simulink library "sm_carousel_lib"  (R2021b)
settings: Solver=ode45  StartTime=0.0  StopTime=10.0  RelTol=1e-3  EnableMultiTasking=on
undefined symbols (not defined in the file): X, Y, Z
libraries: sm_lib x123, $bdroot x16, fl_lib x12, nesl_utility x2
(part 1 of 4)
settings Model: Creator=The MathWorks, Inc.  LastModifiedBy=The MathWorks, Inc.
settings SolverCC: AlgebraicLoopSolver=TrustRegion
settings DataIOCC: LimitDataPoints=on  SaveFormat=Array  ReturnWorkspaceOutputs=off
settings OptimizationCC: ExpressionDepthLimit=2147483647  LifeSpan=inf
settings DebuggingCC: UnderspecifiedInitializationDetection=Classic  MergeDetectMultiDrivingBlocksExec=none  SolverPrmCheckMsg=warning  StateNameClashWarn=warning  SFUnexpectedBacktrackingDiag=warning  SFNoUnconditionalDefaultTransitionDiag=warning  SFExecutionAtInitializationDiag=none  SFMachineParentedDataDiag=warning  ArithmeticOperatorsInVariantConditions=warning
settings HardwareCC: ProdBitPerPointer=32  ProdBitPerSizeT=32  ProdBitPerPtrDiffT=32  ProdLargestAtomicFloat=None  ProdIntDivRoundTo=Undefined  ProdEndianess=Unspecified  ProdWordSize=32  ProdHWDeviceType=32-bit Generic
settings ModelReferenceCC: PropagateSignalLabelsOutOfModel=off
settings SFSimCC: SimUseLocalCustomCode=off  CustomCodeUndefinedFunction=UseInterfaceOnly
settings RTWCC: RTWUseLocalCustomCode=off
settings CodeAppCC: StateflowObjectComments=on
settings GRTTargetCC: TargetLangStandard=C89/C90 (ANSI)
settings ConfigComp: CovMetricSettings=dw  CovSaveCumulativeToWorkspaceVar=on  CovSaveSingleToWorkspaceVar=on  CovExternalEMLEnable=off  CovSFcnEnable=off

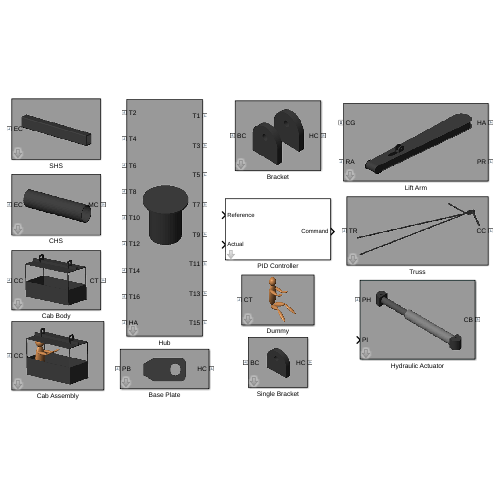
[thumbnail: Simulink's stored preview of the top-level diagram]
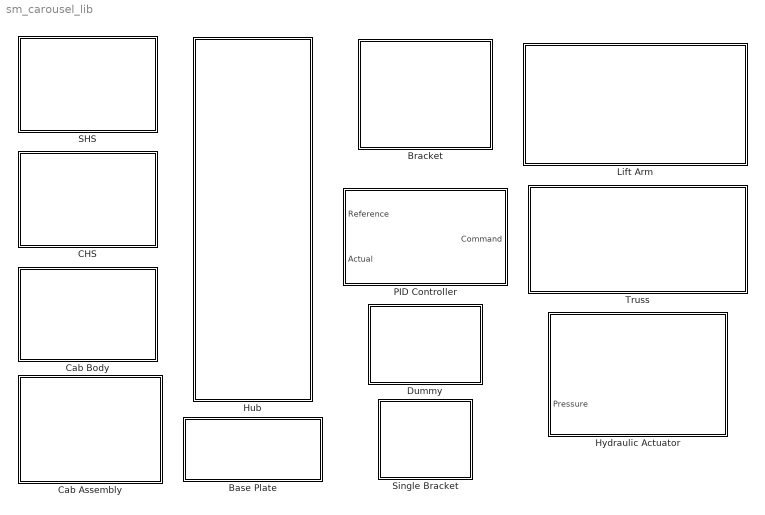
== system sm_carousel_lib ==
  Base Plate : Subsystem  mask(Base Plate){ConnectionDepth=0.1, BasePlateWidth=0.4, BasePlateHeight=0.2, TaperedLength=0.1, rHole=0.05, BasePlateThickness=0.01, HoleOffset=0.3, rho=7800, PlateColor=[0.3 0.3 0.3]}
      mask prompts: ConnectionDepth "Connection Depth (m)"; BasePlateWidth "Plate Width (m)"; BasePlateHeight "Plate Height (m)"; TaperedLength "Tapered Length (m)"; rHole "Hole Radius (m)"; BasePlateThickness "Plate Thickness (m)"; HoleOffset "Hole Offset (m)"; rho "Density (kg/m^3)"; PlateColor "Color [r g b]"
      mask help:
      | This block models a structural element called a Base Plate.
      |
      | It is a utility part designed to serve two purposes:
      | 1) Provide a method to connect the Cab Assembly to the truss via a revolute.
      | 2) To connect the CHS and SHS elements in the Truss block.
      |
      | Attachment points are:
      | 1) The central point of the cross-section at one end of the element (PB).
      | 2) The center of the hole (HC).
      |
      | Click on Help to view a schematic of the Base Plate and its configurable dimension parameters.
      mask init:
      | points = 40;
      | 
      | thetaHole = linspace(pi,-pi,points);
      | 
      | hole = [rHole*cos(thetaHole)+HoleOffset;...
      |     rHole*sin(thetaHole)]';
      | 
      | outerVertices = [0 0;...
      |     0 -0.5*ConnectionDepth;...
      |     TaperedLength -0.5*BasePlateHeight;...
      |     BasePlateWidth -0.5*BasePlateHeight;...
      |     BasePlateWidth 0.5*BasePlateHeight;...
      |     TaperedLength 0.5*BasePlateHeight;...
      |     0 0.5*ConnectionDepth;
      |     0 0];
      |     
      | outer = simmechanics.demohelpers.round_corners(outerVertices,[4 5],rHole,points);
      | 
      | BasePlatePoints = [hole;outer];
      mask Help: web(fullfile(matlabroot,'toolbox','physmod','sm','smdemos','carousel','demohelp','sm_carousel_base_plate.html'));
      mask DialogControl Tab01 Prompt: Dimensions
      mask DialogControl Tab02 Prompt: Material Properties
      mask Display:
      | image(fullfile(matlabroot,'toolbox','physmod','sm','smdemos','carousel','images','sm_carousel_base_plate.png'));
      | port_label('lconn',1,'PB');
      | port_label('rconn',1,'HC');
  Bracket : Subsystem  mask(Bracket){Hbracket=0.75, Wbracket=0.75, Tbracket=0.15, Dbracket=0.8, Hhole=0.5, Rhole=0.075, rhoBracket=7800, bracketColor=[0.3 0.3 0.3]}
      mask prompts: Hbracket "Hbracket (m)"; Wbracket "Wbracket (m)"; Tbracket "Tbracket (m)"; Dbracket "Dbracket (m)"; Hhole "Hhole (m)"; Rhole "Rhole (m)"; rhoBracket "Density (kg/m^3)"; bracketColor "Bracket Color [r g b]"
      mask help:
      | This block models a double-sided bracket.
      |
      | Attachment points are:
      | 1) The base of the bracket centered between the two elements (BC).
      | 2) The central point between the two holes which is configured for Revolute joints (HC).
      |
      | Click on Help to view a schematic of the bracket and its configurable dimension parameters.
      mask init:
      | points = 40;
      | 
      | y = Hbracket - (Wbracket/2);
      | 
      | outerVertices = [0 0;...
      |     Wbracket/2 0;...
      |     Wbracket/2 y;...
      |     Wbracket/2 Hbracket;...
      |     -Wbracket/2 Hbracket;...
      |     -Wbracket/2 y;...
      |     -Wbracket/2 0;...
      |     0 0];
      | 
      | outer = simmechanics.demohelpers.round_corners(outerVertices,[4 5],Wbracket/2,points);
      | 
      | thetaHole = linspace(1.5*pi,-0.5*pi,points);
      | hole = [Rhole*cos(thetaHole);...
      |     Rhole*sin(thetaHole)+Hhole]';
      | 
      | bracketPoints = [hole;outer];
      mask Help: web(fullfile(matlabroot,'toolbox','physmod','sm','smdemos','carousel','demohelp','sm_carousel_bracket.html'));
      mask DialogControl Tab01 Prompt: Dimensions
      mask DialogControl Tab02 Prompt: Material Properties
      mask Display:
      | image(fullfile(matlabroot,'toolbox','physmod','sm','smdemos','carousel','images','sm_carousel_bracket.png'));
      | port_label('lconn',1,'BC');
      | port_label('rconn',1,'HC');
  CHS : Subsystem  mask(Circular Hollow Section (CHS)){PinOuterRadius=0.1, PinThickness=0.01, PinDepth=1, rhoPin=7800, PinColor=[0.3 0.3 0.3]}
      mask prompts: PinOuterRadius "Outer Radius (m)"; PinThickness "Thickness (m)"; PinDepth "Length (m)"; rhoPin "Density (kg/m^3)"; PinColor "Color [r g b]"
      mask help:
      | This block models a Circular Hollow Section structural element.
      |
      | Attachment points are:
      | 1) The central point of the cross-section at one end of the element (EC).
      | 2) The central point of the cross-section at the center of the element (MC).
      |
      | Click on Help to view a schematic of the CHS and its configurable dimension parameters.
      mask init:
      | %%% Pin
      | 
      | points = 40;
      | 
      | PinInnerRadius = PinOuterRadius-PinThickness;
      | 
      | thetaInner = linspace(2*pi,0,points);
      | inner = [PinInnerRadius*cos(thetaInner);...
      |     PinInnerRadius*sin(thetaInner)]';
      | 
      | thetaOuter = fliplr(thetaInner);
      | outer = [PinOuterRadius*cos(thetaOuter);...
      |     PinOuterRadius*sin(thetaOuter)]';
      | 
      | Pin = [inner;outer];
      | 
      | %%% End Pin
      mask Help: web(fullfile(matlabroot,'toolbox','physmod','sm','smdemos','carousel','demohelp','sm_carousel_CHS.html'));
      mask DialogControl Tab01 Prompt: Dimensions
      mask DialogControl Tab02 Prompt: Material Properties
      mask Display:
      | image(fullfile(matlabroot,'toolbox','physmod','sm','smdemos','carousel','images','sm_carousel_CHS.png'));
      | port_label('lconn',1,'EC');
      | port_label('rconn',1,'MC');
  Cab Assembly : Subsystem  mask(Cab Assembly){CabLength=1.5, CabWidth=0.75, CabPlateThickness=0.02, CabBodyConnW=0.05, CabBodyConnH=0.07, CabWindowHeight=0.5, SpacerThickness=0.02, CabTubDepth=0.45, RP_CD=0.1, RP_W=0.23, RP_H=0.18, RP_TL=0.07, RP_HR=0.04, RP_PT=0.01, RP_HO=0.15, DummyHeight=1.83, DummyDensity=950, rhoCab=7800, CabColor=[0.3 0.3 0.3]}
      mask prompts: CabLength "Cab Length (m)"; CabWidth "Cab Width (m)"; CabPlateThickness "Cab Plate Thickness (m)"; CabBodyConnW "Cab Body Connector Width (m)"; CabBodyConnH "Cab Body Connector Height (m)"; CabWindowHeight "Cab Window Height (m)"; SpacerThickness "Cab Window Column Thickness (m)"; CabTubDepth "Cab Tub Depth (m)"; RP_CD "Connection Depth (m)"; RP_W "Plate Width (m)"; RP_H "Plate Height (m)"; RP_TL "Tapered Length (m)"; RP_HR "Hole Radius (m)"; RP_PT "Plate Thickness (m)"; RP_HO "Hole Offset (m)"; DummyHeight "Dummy Height (m)"; DummyDensity "Dummy Density (kg/m^3)"; rhoCab "Cab Density (kg/m^3)"; CabColor "Cab Color [r g b]"
      mask help:
      | This block models the Carousel Cab Assembly.
      |
      | The block includes: 2x Base Plate, 1x Cab Body, 1x Dummy.
      |
      | Attachment point is the central point between the holes of the two revolute plates.
      |
      | Click on Help to view a schematic of the Cab Assembly. The configurable dimensions are not shown. Refer to the Help of the individual parts for more information.
      mask Help: web(fullfile(matlabroot,'toolbox','physmod','sm','smdemos','carousel','demohelp','sm_carousel_cab_assembly.html'));
      mask DialogControl Tab01 Prompt: Cab Body Main
      mask DialogControl Tab02 Prompt: Cab Body Revolute Plate
      mask DialogControl Tab03 Prompt: Dummy
      mask DialogControl Tab04 Prompt: Material Properties
      mask Display:
      | image(fullfile(matlabroot,'toolbox','physmod','sm','smdemos','carousel','images','sm_carousel_cab_assembly.png'));
      | port_label('lconn',1,'CC');
  Cab Body : Subsystem  mask(Cab Body){CabLength=1.5, CabWidth=0.75, PlateThickness=0.02, ConnectorWidth=0.05, ConnectorHeight=0.07, SpacerHeight=0.5, SpacerThickness=0.02, TubDepth=0.45, RP_CD=0.1, RP_W=0.23, RP_H=0.18, RP_TL=0.07, RP_HR=0.04, RP_PT=0.01, RP_HO=0.15, rhoCab=7800, CabColor=[0.3 0.3 0.3]}
      mask prompts: CabLength "Cab Length (m)"; CabWidth "Cab Width (m)"; PlateThickness "Cab Plate Thickness (m)"; ConnectorWidth "Connector Width (m)"; ConnectorHeight "Connector Height (m)"; SpacerHeight "Spacer Height (m)"; SpacerThickness "Spacer Thickness (m)"; TubDepth "Tub Depth (m)"; RP_CD "Connection Depth (m)"; RP_W "Plate Width (m)"; RP_H "Plate Height (m)"; RP_TL "Tapered Length (m)"; RP_HR "Hole Radius (m)"; RP_PT "Plate Thickness (m)"; RP_HO "Hole Offset (m)"; rhoCab "Cab Density (kg/m^3)"; CabColor "Cab Color [r g b]"
      mask help:
      | This block models the Carousel Cab Body.
      |
      | Attachment points are:
      | 1) The central point of the cross-section of the connection element which is attached to the roof element (CC).
      | 2) Fixed location in the cab interior to attach a Carousel Dummy (CT).
      |
      | Click on Help to view a schematic of the Cab Body and its configurable dimension parameters. The Revolute Plates are shown in red and the dimensions are not shown for clarity. Refer to the Help of the Base Plate for more information.
      mask init:
      | % Revolute Plates
      | 
      | CabRotatePlateOffset = 0.33*CabLength; % m
      | CabConnectorOffsetFromPlate = [ConnectorHeight/2-RP_HO 0 0];
      | 
      | % Connector Dimensions
      | 
      | Connector = [CabLength ConnectorWidth ConnectorHeight];
      | ConnectorOffsetFromRoof = (ConnectorHeight + PlateThickness)/2;
      | 
      | % Roof Dimensions
      | 
      | Roof = [CabLength CabWidth PlateThickness];
      | RoofOffsetFromCabBodyCenter = SpacerHeight+PlateThickness/2;
      | 
      | % Spacer Dimensions
      | 
      | Spacer = [SpacerThickness SpacerThickness SpacerHeight];
      | 
      | SpacerOffsetFromCenter1 = [CabLength/2-SpacerThickness/2 ...
      |     CabWidth/2-SpacerThickness/2 ...
      |     SpacerHeight/2];
      | 
      | SpacerOffsetFromCenter2 = [-(CabLength/2-SpacerThickness/2) ...
      |     CabWidth/2-SpacerThickness/2 ...
      |     SpacerHeight/2];
      | 
      | SpacerOffsetFromCenter3 = [-(CabLength/2-SpacerThickness/2) ...
      |     -(CabWidth/2-SpacerThickness/2) ...
      |     SpacerHeight/2];
      | 
      | SpacerOffsetFromCenter4 = [CabLength/2-SpacerThickness/2 ...
      |     -(CabWidth/2-SpacerThickness/2) ...
      |     SpacerHeight/2];
      | 
      | % Tub Dimensions
      | 
      | TubCenterFromCabBodyCenter = TubDepth/2;
      | 
      | TubSide = [TubDepth PlateThickness CabLength];
      | TubFront = [PlateThickness CabWidth TubDepth];
      | TubBottom = [CabLength CabWidth PlateThickness];
      | 
      | TubSideFromCenter = (CabWidth-PlateThickness)/2;
      | TubFrontFromCenter = (CabLength-PlateThickness)/2;
      | TubBottomFromCenter = (TubDepth-PlateThickness)/2;
      | 
      | % Person Center
      | 
      | PersonCenter = [-0.4*CabLength  0 -0.15*TubDepth];
      mask Help: web(fullfile(matlabroot,'toolbox','physmod','sm','smdemos','carousel','demohelp','sm_carousel_cab_body.html'));
      mask DialogControl Tab01 Prompt: Cab Body
      mask DialogControl Tab02 Prompt: Revolute Plate
      mask DialogControl Tab03 Prompt: Material Properties
      mask Display:
      | image(fullfile(matlabroot,'toolbox','physmod','sm','smdemos','carousel','images','sm_carousel_cab_body.png'));
      | port_label('lconn',1,'CC');
      | port_label('rconn',1,'CT');
  Dummy : Subsystem  mask(Dummy){height=1.83, personDensity=950}
      mask prompts: height "Dummy Height (m)"; personDensity "Dummy Density (kg/m^3)"
      mask help:
      | This block models a Test Dummy for the Carousel.
      |
      | The attachment point is the central point of the Torso (CT).
      |
      | Click on Help to view a schematic of the Dummy and its configurable dimension parameters.
      mask init:
      | % Person initialization
      | % http://www.mech.utah.edu/ergo/pages/Educational/safety_modules/ctd-anthropometry/index.html
      | 
      | personColor = [244 164 96]/255;
      | 
      | %%
      | lTorso = (0.52-0.13)*height;
      | rTorso = [0.05*height 0.5*0.174*height lTorso/2];
      | %%
      | rHead = 0.5*0.13*height;
      | headFromTorso = 0.5*rHead+0.5*lTorso;
      | %%
      | lArmUpper = 0.186*height;
      | rArmUpper = [0.02*height 0.03*height lArmUpper/2];
      | %%
      | lArmLower = 0.156*height;
      | rArmLower = [0.015*height 0.02*height lArmLower/2];
      | armLowerRotation = -30; % deg
      | %%
      | lLegUpper = (0.53-0.285)*height;
      | rLegUpper = [0.03*height 0.04*height lLegUpper/2];
      | legUpperRotation1 = -20; % deg
      | legUpperRotation2 = -15; % deg
      | %%
      | lLegLower = 0.25*height;
      | rLegLower = [0.02*height 0.03*height lLegLower/2];
      | legLowerRotation = 40; % deg
      | %%
      | leftLegFromTorso = [0 0.3*rTorso(2) -0.5*lTorso];
      | rightLegFromTorso = [0 -0.3*rTorso(2) -0.5*lTorso];
      | 
      | leftArmFromTorso = [0 0.7*rTorso(2) 0.25*lTorso];
      | rightArmFromTorso = [0 -0.7*rTorso(2) 0.25*lTorso];
      mask Help: web(fullfile(matlabroot,'toolbox','physmod','sm','smdemos','carousel','demohelp','sm_carousel_dummy.html'));
      mask Display:
      | image(fullfile(matlabroot,'toolbox','physmod','sm','smdemos','carousel','images','sm_carousel_dummy.png'));
      | port_label('lconn',1,'CT');
  Hub : Subsystem  mask(Hub){HubOuterRadius=0.5, HubThickness=0.01, HubDepth=1.18, HubCapRadius=0.7, HubCapThickness=0.05, nCabs=16, rho=7800, HubColor=[0.3 0.3 0.3]}
      mask prompts: HubOuterRadius "Outer Radius (m)"; HubThickness "Thickness (m)"; HubDepth "Depth (m)"; HubCapRadius "Cap Radius (m)"; HubCapThickness "Cap Thickness (m)"; nCabs "Number of Cabs"; rho "Density (kg/m^3)"; HubColor "Color [r g b]"
      mask help:
      | This block models the Hub for the Carousel wheel assembly.
      |
      | The block includes: 1x CHS
      |
      | Attachment points are:
      | 1) Center of the cross-section at the base of the Hub (HA).
      | 2) Frames at perimeter of Hub to attach 16 Truss assemblies (T#).
      |
      | Click on Help to view a schematic of the Hub Assembly and its configurable dimension parameters.
      | N.B.: Parts in the help are shown in different colors to aid the clarity of the schematic.
      mask init:
      | thetaCab = 360/(nCabs);
      | thetaCabs = thetaCab*(0:nCabs-1);
      mask Help: web(fullfile(matlabroot,'toolbox','physmod','sm','smdemos','carousel','demohelp','sm_carousel_hub.html'));
      mask DialogControl Tab01 Prompt: Hub
      mask DialogControl Tab02 Prompt: Cap
      mask DialogControl Tab03 Prompt: Cabs
      mask DialogControl Tab04 Prompt: Material Properties
      mask Display:
      | image(fullfile(matlabroot,'toolbox','physmod','sm','smdemos','carousel','images','sm_carousel_hub.png'));
      | port_label('rconn',1,'T1');
      | port_label('rconn',2,'T3');
      | port_label('rconn',3,'T5');
      | port_label('rconn',4,'T7');
      | port_label('rconn',5,'T9');
      | port_label('rconn',6,'T11');
      | port_label('rconn',7,'T13');
      | port_label('rconn',8,'T15');
      | 
      | port_label('lconn',1,'T2');
      | port_label('lconn',2,'T4');
      | port_label('lconn',3,'T6');
      | port_label('lconn',4,'T8');
      | port_label('lconn',5,'T10');
      | port_label('lconn',6,'T12');
      | port_label('lconn',7,'T14');
      | port_label('lconn',8,'T16');
      | port_label('lconn',9,'HA');
  Hydraulic Actuator : Subsystem  mask(Hydraulic Actuator){Lcyl=1.4, Rcyl=0.11, Lbase=0.2, Wbase=0.24, Rbp=0.02, Lpist=1.4, Rpist=0.1, Whead=0.24, Lhead=0.18, Rhp=0.025, cylColor=[0.6 0.6 0.6], rhoCyl=7800, pistColor=[0.4 0.4 0.4], rhoPist=7800, connColor=[0.3 0.3 0.3], rhoConn=7800}
      mask prompts: Lcyl "Lcyl (m)"; Rcyl "Rcyl (m)"; Lbase "Lbase (m)"; Wbase "Wbase(m)"; Rbp "Rbp (m)"; Lpist "Lpist (m)"; Rpist "Rpist (m)"; Whead "Whead (m)"; Lhead "Lhead (m)"; Rhp "Rhp (m)"; cylColor "Cylinder Color"; rhoCyl "Cylinder Density (kg/m^3)"; pistColor "Piston Color"; rhoPist "Piston Density (kg/m^3)"; connColor "Connector Color"; rhoConn "Connector Density (kg/m^3)"
      mask help:
      | This block models a hydraulic actuator.
      |
      | The block includes: 2x Single Bracket, 1x CHS.
      |
      | Positive piston displacement is outward motion, and negative piston displacement is inward motion.
      |
      | Attachment points are:
      | 1) Center of the Cylinder base bracket hole (CB).
      | 2) Center of the Piston Head bracket hole (PH).
      | Both attachment points are configured for Revolute joints.
      |
      | The Simulink Signal input port supplies a Pressure value P (Bar) to a Simscape hydraulic network.
      |
      | Click on Help to view a schematic of the hydraulic actuator, its configurable dimension parameters.
      mask init:
      | cylThickness = Rcyl - Rpist;
      mask Help: web(fullfile(matlabroot,'toolbox','physmod','sm','smdemos','carousel','demohelp','sm_carousel_actuator.html'));
      mask DialogControl Tab01 Prompt: Cylinder
      mask DialogControl Tab02 Prompt: Piston
      mask DialogControl Tab03 Prompt: Material Properties
      mask Display:
      | image(fullfile(matlabroot,'toolbox','physmod','sm','smdemos','carousel','images','sm_carousel_actuator.png'));
      | port_label('lconn',1,'PH');
      | port_label('rconn',1,'CB');
      | port_label('input',1,'PI');
  Lift Arm : Subsystem  mask(Lift Arm){LiftArmLength=6.5, rootWidth=0.7, ArmRadius=0.55, LiftArmDepth=0.5, LiftArmLip=0.05, plateThickness=0.02, Hbracket=0.4, Wbracket=0.4, Tbracket=0.05, Dbracket=0.3, Hhole=0.2, Rhole=0.04, PistonBracketOffset=4.6, TopHoleOffset=4.78, TopHoleW=0.24, TopHoleL=0.65, BottomHoleOffset=5.12, BottomHoleW=0.24, BottomHoleL=0.95, rhoLiftArm=7800, LiftArmColor=[0.3 0.3 0.3]}
      mask prompts: LiftArmLength "Arm Length (m)"; rootWidth "Arm Root Width (m)"; ArmRadius "Arm Radius (m)"; LiftArmDepth "Arm Depth (m)"; LiftArmLip "Arm Lip (m)"; plateThickness "Thickness (m)"; Hbracket "Height (m)"; Wbracket "Width (m)"; Tbracket "Thickness (m)"; Dbracket "Depth (m)"; Hhole "Hole Offset (m)"; Rhole "Hole Radius (m)"; PistonBracketOffset "Bracket Offset (m)"; TopHoleOffset "Hole Offset (m)"; TopHoleW "Hole Width (m)"; TopHoleL "Hole Length (m)"; BottomHoleOffset "Hole Offset (m)"; BottomHoleW "Hole Width (m)"; BottomHoleL "Hole Length (m)"; rhoLiftArm "Density (kg/m^3)"; LiftArmColor "Color [r g b]"
      mask help:
      | This block models the Lift Arm for the Carousel.
      |
      | The block includes: 1x Bracket
      |
      | The holes in the top and bottom plates provide access to the bracket for connecting a hydraulic cylinder.
      |
      | Attachment points are:
      | 1) Frame attached to bottom plate for contact point with the ground (CP).
      | 2) Central axis of End Cap perpendicular to the bearings (RA).
      | 3) Central axis perpendicular to the bracket holes (PR).
      | 4) Frame attached to top plate for joint with the wheel hub (HA).
      |
      | Click on Help to view a schematic of the Lift Arm and its configurable dimension parameters.
      | N.B.:
      | a) See help for the Bracket for configurable dimensions of the Actuator Bracket.
      | b) Top and bottom plates are shown in different colors in the help to show the holes clearly.
      mask init:
      | points = 20;
      | 
      | %%% TOP AND BOTTOM PLATE %%%
      | 
      | plateOffset = LiftArmDepth/2;
      | 
      | plateOuterVertices = [ArmRadius 0;...
      |     ArmRadius ArmRadius;...
      |     -ArmRadius ArmRadius;...
      |     -ArmRadius 0;...
      |     -rootWidth/2 -LiftArmLength;...
      |     rootWidth/2 -LiftArmLength;...
      |     ArmRadius 0];
      | 
      | plateOuter = simmechanics.demohelpers.round_corners(plateOuterVertices,[2 3],ArmRadius,points);
      | 
      | % Top Plate
      | 
      | topHoleVertices = [0.5*TopHoleW -TopHoleOffset;...
      |     0.5*TopHoleW -TopHoleOffset-TopHoleL;...
      |     -0.5*TopHoleW -TopHoleOffset-TopHoleL;...
      |     -0.5*TopHoleW -TopHoleOffset];
      | 
      | topHole = simmechanics.demohelpers.round_corners(topHoleVertices,[1 2 3 4],0.5*TopHoleW,points);
      | 
      | TopPlate = [topHole;plateOuter];
      | 
      | % Bottom Plate
      | 
      | bottomHoleVertices = [0.5*BottomHoleW -BottomHoleOffset;...
      |     0.5*BottomHoleW -BottomHoleOffset-BottomHoleL;...
      |     -0.5*BottomHoleW -BottomHoleOffset-BottomHoleL;...
      |     -0.5*BottomHoleW -BottomHoleOffset];
      | 
      | bottomHole = simmechanics.demohelpers.round_corners(bottomHoleVertices,[1 2 3 4],0.5*BottomHoleW,points);
      | 
      | BottomPlate = [bottomHole;plateOuter];
      | 
      | %%% Arm Bracing
      | 
      | rBracingOuter = ArmRadius - LiftArmLip;
      | rBracingInner = rBracingOuter - plateThickness;
      | bracingRootOuter = rootWidth/2 - LiftArmLip;
      | bracingRootInner = bracingRootOuter - plateThickness;
      | 
      | bracingVertices = [rBracingOuter 0;...
      |     rBracingOuter rBracingOuter;...
      |     -rBracingOuter rBracingOuter;...
      |     -rBracingOuter 0;...
      |     -bracingRootOuter -LiftArmLength;...
      |     -bracingRootInner -LiftArmLength;...
      |     -rBracingInner 0;...
      |     -rBracingInner rBracingInner;...
      |     rBracingInner rBracingInner;...
      |     rBracingInner 0;...
      |     bracingRootInner -LiftArmLength;...
      |     bracingRootOuter -LiftArmLength];
      | 
      | armBracing = simmechanics.demohelpers.round_corners(bracingVertices,[2 3 8 9],[rBracingOuter rBracingOuter rBracingInner rBracingInner],points);
      | 
      | %%% END CAP %%%
      | 
      | % End Cap
      | 
      | rCapInner = LiftArmDepth/2-0.5*plateThickness;
      | rCapOuter = rCapInner+plateThickness;
      | 
      | capVertices = [0 rCapOuter;...
      |     -rCapOuter rCapOuter;...
      |     -rCapOuter -rCapOuter;...
      |     0 -rCapOuter;...
      |     0 -rCapInner;...
      |     -rCapInner -rCapInner;...
      |     -rCapInner rCapInner;...
      |     0 rCapInner];
      | 
      | cap = simmechanics.demohelpers.round_corners(capVertices,[2 3 6 7],[rCapOuter rCapOuter rCapInner rCapInner],points);
      | 
      | % Bearing
      | 
      | rBearing = rCapOuter+LiftArmLip;
      | 
      | %%% ACTUATOR BRACKET %%%
      | 
      | bracketOffset = [0 -PistonBracketOffset LiftArmDepth/2];
      mask Help: web(fullfile(matlabroot,'toolbox','physmod','sm','smdemos','carousel','demohelp','sm_carousel_lift_arm.html'));
      mask DialogControl Tab01 Prompt: Arm Main
      mask DialogControl Tab02 Prompt: Actuator Bracket
      mask DialogControl Tab03 Prompt: Top Plate
      mask DialogControl Tab04 Prompt: Bottom Plate
      mask DialogControl Tab05 Prompt: Material Properties
      mask Display:
      | image(fullfile(matlabroot,'toolbox','physmod','sm','smdemos','carousel','images','sm_carousel_lift_arm.png'));
      | port_label('lconn',1,'CG');
      | port_label('lconn',2,'RA');
      | port_label('rconn',1,'HA');
      | port_label('rconn',2,'PR');
  PID Controller : Subsystem  mask(PID Controller){Kp=5e7, Ki=1e5, Kd=0, N=5}
      mask help:
      | This block models a PID controller using Simulink blocks.
      |
      | This block takes in a reference signal and actual signal to calculate a control command.
      |
      | Click on Help to view the equation that is solved.
      mask Help: web(fullfile(matlabroot,'toolbox','physmod','sm','smdemos','carousel','demohelp','sm_carousel_PID.html'));
  SHS : Subsystem  mask(Square Hollow Section (SHS)){width=0.1, thickness=0.01, length=1, rho_SHS=7800, SHSColor=[0.3 0.3 0.3]}
      mask prompts: width "Width (m)"; thickness "Thickness (m)"; length "Length (m)"; rho_SHS "Density (kg/m^3)"; SHSColor "Color [r g b]"
      mask help:
      | This block models a Square Hollow Section structural element.
      |
      | Attachment point is the End Center of the cross-section at one end of the element (EC).
      |
      | Click on Help to view a schematic of the SHS and its configurable dimension parameters.
      mask init:
      | points = 20;
      | 
      | CornerOffset = 0.5*width-thickness;
      | 
      | outerVertices = [0.5*width 0.5*width;...
      |     -0.5*width 0.5*width;...
      |     -0.5*width -0.5*width;...
      |     0.5*width -0.5*width];
      | 
      | outer = simmechanics.demohelpers.round_corners(outerVertices,[1 2 3 4],thickness,points);
      | 
      | inner = [CornerOffset CornerOffset;...
      |     CornerOffset -CornerOffset;...
      |     -CornerOffset -CornerOffset;...
      |     -CornerOffset CornerOffset;...
      |     CornerOffset CornerOffset];
      | 
      | SHS_points = [inner; outer; outer(1,:)];
      mask Help: web(fullfile(matlabroot,'toolbox','physmod','sm','smdemos','carousel','demohelp','sm_carousel_SHS.html'));
      mask DialogControl Tab01 Prompt: Dimensions
      mask DialogControl Tab02 Prompt: Material Properties
      mask Display:
      | image(fullfile(matlabroot,'toolbox','physmod','sm','smdemos','carousel','images','sm_carousel_SHS.png'));
      | port_label('lconn',1,'EC');
  Single Bracket : Subsystem  mask(Single Bracket){Hbracket=0.75, Wbracket=0.75, Tbracket=0.15, Hhole=0.5, Rhole=0.075, rho=7780, bracketColor=[0.3 0.3 0.3]}
      mask prompts: Hbracket "Hbracket (m)"; Wbracket "Wbracket (m)"; Tbracket "Tbracket (m)"; Hhole "Hhole (m)"; Rhole "Rhole (m)"; rho "Density (kg/m^3)"; bracketColor "Bracket Color"
      mask help:
      | This block models a single element bracket.
      |
      | This part is used exclusively in the Hydraulic Actuator.
      |
      | Attachment points are:
      | 1) The central point of the base (BC).
      | 2) The center point of the hole, which is configured for Revolute joints (HC).
      |
      | Click on Help to view a schematic of the bracket, its configurable dimension parameters and attachment points (in red).
      mask init:
      | points = 40;
      | 
      | y = Hbracket - (Wbracket/2);
      | 
      | outerVertices = [0 0;...
      |     Wbracket/2 0;...
      |     Wbracket/2 y;...
      |     Wbracket/2 Hbracket;...
      |     -Wbracket/2 Hbracket;...
      |     -Wbracket/2 y;...
      |     -Wbracket/2 0;...
      |     0 0];
      | 
      | outer = simmechanics.demohelpers.round_corners(outerVertices,[4 5],Wbracket/2,points);
      | 
      | thetaHole = linspace(1.5*pi,-0.5*pi,points);
      | 
      | hole = [Rhole*cos(thetaHole);...
      |     Rhole*sin(thetaHole)+Hhole]';
      | 
      | bracketPoints = [hole;outer];
      mask Help: web(fullfile(matlabroot,'toolbox','physmod','sm','smdemos','carousel','demohelp','sm_carousel_single_bracket.html'));
      mask DialogControl Tab01 Prompt: Dimensions
      mask DialogControl Tab02 Prompt: Material Properties
      mask Display:
      | image(fullfile(matlabroot,'toolbox','physmod','sm','smdemos','carousel','images','sm_carousel_single_bracket.png'));
      | port_label('lconn',1,'BC');
      | port_label('rconn',1,'HC');
  Truss : Subsystem  mask(Truss Assembly){RootDepth=0.8, TrussLength=5, MemberWidth=0.05, MemberThickness=0.01, BraceLength=1.72, BraceAngle=99, EPConnectionDepth=0.1, EPWidth=0.4, EPHeight=0.2, EPTaperedLength=0.1, EPHoleRadius=0.04, EPThickness=0.01, EPHoleOffset=0.3, PinAngle=9, PinOuterRadius=0.04, PinThickness=0.01, PinLength=1.81, rhoTruss=7800, TrussColor=[0.3 0.3 0.3]}
      mask prompts: RootDepth "Root Depth (m)"; TrussLength "Truss Length (m)"; MemberWidth "Member Width (m)"; MemberThickness "Member Thickness (m)"; BraceLength "Brace Length (m)"; BraceAngle "Brace Angle (deg)"; EPConnectionDepth "Connection Depth (m)"; EPWidth "Plate Width (m)"; EPHeight "Plate Height (m)"; EPTaperedLength "Tapered Length (m)"; EPHoleRadius "Hole Radius (m)"; EPThickness "Plate Thickness (m)"; EPHoleOffset "Hole Offset (m)"; PinAngle "Pin Angle (deg)"; PinOuterRadius "Pin Outer Radius (m)"; PinThickness "Pin Thickness (m)"; PinLength "Pin Length (m)"; rhoTruss "Density (kg/m^3)"; TrussColor "Color [r g b]"
      mask help:
      | This block models an element of the spoke and rim of the Carousel wheel.
      |
      | The block includes: 3x SHS, 1x CHS, 1x Base Plate.
      |
      | Attachment points are:
      | 1) The central point at the truss root to connect with the Carousel Hub (TR).
      | 2) The mid-point of the truss pin to locate a cab assembly (CC).
      |
      | Click on Help to view a schematic of the Truss Assembly and its configurable dimension parameters.
      | N.B.:
      | a) Refer to the Help of the Base Plate for the End Plate configurable dimensions.
      | b) The 'Member Width' and 'Member Thickness' refer to the configurable dimensions of the three SHS elements.
      mask init:
      | rotateX = atand(RootDepth/TrussLength);
      | trussSHSLength = sqrt(TrussLength^2+(0.5*RootDepth)^2)+MemberWidth;
      | trussEnd = [0 0 -(TrussLength-0.3*MemberWidth)];
      mask Help: web(fullfile(matlabroot,'toolbox','physmod','sm','smdemos','carousel','demohelp','sm_carousel_truss.html'));
      mask DialogControl Tab01 Prompt: Truss
      mask DialogControl Tab02 Prompt: End Plate
      mask DialogControl Tab03 Prompt: Cab Pin
      mask DialogControl Tab04 Prompt: Material Properties
      mask Display:
      | image(fullfile(matlabroot,'toolbox','physmod','sm','smdemos','carousel','images','sm_carousel_truss.png'));
      | port_label('lconn',1,'TR');
      | port_label('rconn',1,'CC');

== system sm_carousel_lib/Base Plate ==
  Base Plate : sm_lib/Body Elements/Extruded Solid  GraphicAmbientColor=[0.15 0.15 0.15 1.0]  BasedOnType=Density  CenterOfMass=[0 0 0]  CenterOfMassUnits=m  GraphicDiffuseColor=PlateColor  ExportConvexHullGeometry=off  ExtrusionCrossSection=BasePlatePoints  ExtrusionCrossSectionUnits=m  Density=rho  DensityUnits=kg/(m^3)  DoExposeReferenceFrame=on  GraphicEmissiveColor=[0.0 0.0 0.0 1.0]  ExportEntireGeometry=off  ExtrusionLength=BasePlateThickness  ExtrusionLengthUnits=m  ExtrusionType=General  SerializedFrames=<Frames/>  MarkerShape=Sphere  MarkerSize=10  GraphicType=FromGeometry  InertiaType=CalculateFromGeometry  Mass=1  MassUnits=kg  MomentsOfInertia=[1 1 1]  MomentsOfInertiaUnits=kg*m^2  PolygonNumSides=3  GraphicOpacity=1.0  PolygonOuterRadius=1  PolygonOuterRadiusUnits=m  ProductsOfInertia=[0 0 0]  ProductsOfInertiaUnits=kg*m^2  GraphicShininess=75  GraphicSpecularColor=[0.5 0.5 0.5 1.0]  GraphicVisPropType=SimpleVisualProperties
  Base to Hole Center XForm : sm_lib/Frames and Transforms/Rigid Transform  TranslationMethod=StandardAxis  TranslationStandardOffset=HoleOffset  TranslationLengthUnit=m  TranslationStandardAxis=+X  TranslationCartesianOffset=[0 0 0]  TranslationROffset=0  TranslationROffsetUnits=m  TranslationZOffset=0  TranslationZOffsetUnits=m  TranslationThetaOffset=0  TranslationThetaOffsetUnits=deg  RotationMethod=None  RotationAngleUnits=deg  RotationStandardAxis=+Z  RotationAngle=0  RotationArbitraryAxis=[0 0 1]  FollAlignAxisA=+X  BaseAlignAxisA=+Y  FollAlignAxisB=+Y  BaseAlignAxisB=+Z  RotationSequenceAxes=FollowerAxes  RotationSequence=XYX  RotationSequenceAngles=[0 0 0]  RotationSequenceAnglesUnits=deg  RotationMatrix=[1 0 0; 0 1 0; 0 0 1]
  Plate Base : PMIOPort  Side=Left
  Hole Center : PMIOPort  Port=2  Side=Right
  connections:
  Plate Base/RConn1 -- Base to Hole Center XForm/LConn1 -- Base Plate/RConn1
  Base to Hole Center XForm/RConn1 -- Hole Center/RConn1

== system sm_carousel_lib/Bracket ==
  Base Cebter to Hole XForm : sm_lib/Frames and Transforms/Rigid Transform  TranslationMethod=StandardAxis  TranslationStandardOffset=Hhole  TranslationLengthUnit=m  TranslationStandardAxis=+Z  TranslationCartesianOffset=[0 (Dbracket-Tbracket)/2 Hbracket/2]  TranslationROffset=0  TranslationROffsetUnits=m  TranslationZOffset=0  TranslationZOffsetUnits=m  TranslationThetaOffset=0  TranslationThetaOffsetUnits=deg  RotationMethod=StandardAxis  RotationAngleUnits=deg  RotationStandardAxis=+X  RotationAngle=90  RotationArbitraryAxis=[0 0 1]  FollAlignAxisA=+X  BaseAlignAxisA=+Y  FollAlignAxisB=+Y  BaseAlignAxisB=+Z  RotationSequenceAxes=FollowerAxes  RotationSequence=XYX  RotationSequenceAngles=[0 0 0]  RotationSequenceAnglesUnits=deg  RotationMatrix=[1 0 0; 0 1 0; 0 0 1]
  Base Center Frame : sm_lib/Frames and Transforms/Reference Frame
  Base Center to Left Bracket XForm : sm_lib/Frames and Transforms/Rigid Transform  TranslationMethod=StandardAxis  TranslationStandardOffset=(Dbracket-Tbracket)/2  TranslationLengthUnit=m  TranslationStandardAxis=-Y  TranslationCartesianOffset=[0 0 0]  TranslationROffset=0  TranslationROffsetUnits=m  TranslationZOffset=0  TranslationZOffsetUnits=m  TranslationThetaOffset=0  TranslationThetaOffsetUnits=deg  RotationMethod=StandardAxis  RotationAngleUnits=deg  RotationStandardAxis=+X  RotationAngle=90  RotationArbitraryAxis=[0 0 1]  FollAlignAxisA=+X  BaseAlignAxisA=+Y  FollAlignAxisB=+Y  BaseAlignAxisB=+Z  RotationSequenceAxes=FollowerAxes  RotationSequence=XYX  RotationSequenceAngles=[0 0 0]  RotationSequenceAnglesUnits=deg  RotationMatrix=[1 0 0; 0 1 0; 0 0 1]
  Base Center to Right Bracket XForm : sm_lib/Frames and Transforms/Rigid Transform  TranslationMethod=StandardAxis  TranslationStandardOffset=(Dbracket-Tbracket)/2  TranslationLengthUnit=m  TranslationStandardAxis=+Y  TranslationCartesianOffset=[0 (Dbracket-Tbracket)/2 Hbracket/2]  TranslationROffset=0  TranslationROffsetUnits=m  TranslationZOffset=0  TranslationZOffsetUnits=m  TranslationThetaOffset=0  TranslationThetaOffsetUnits=deg  RotationMethod=StandardAxis  RotationAngleUnits=deg  RotationStandardAxis=+X  RotationAngle=90  RotationArbitraryAxis=[0 0 1]  FollAlignAxisA=+X  BaseAlignAxisA=+Y  FollAlignAxisB=+Y  BaseAlignAxisB=+Z  RotationSequenceAxes=FollowerAxes  RotationSequence=XYX  RotationSequenceAngles=[0 0 0]  RotationSequenceAnglesUnits=deg  RotationMatrix=[1 0 0; 0 1 0; 0 0 1]
  Left Bracket : sm_lib/Body Elements/Extruded Solid  GraphicAmbientColor=[0.15 0.15 0.15 1.0]  BasedOnType=Density  CenterOfMass=[0 0 0]  CenterOfMassUnits=m  GraphicDiffuseColor=bracketColor  ExportConvexHullGeometry=off  ExtrusionCrossSection=bracketPoints  ExtrusionCrossSectionUnits=m  Density=rhoBracket  DensityUnits=kg/(m^3)  DoExposeReferenceFrame=on  GraphicEmissiveColor=[0.0 0.0 0.0 1.0]  ExportEntireGeometry=off  ExtrusionLength=Tbracket  ExtrusionLengthUnits=m  ExtrusionType=General  SerializedFrames=<Frames/>  MarkerShape=Sphere  MarkerSize=10  GraphicType=FromGeometry  InertiaType=CalculateFromGeometry  Mass=1  MassUnits=kg  MomentsOfInertia=[1 1 1]  MomentsOfInertiaUnits=kg*m^2  PolygonNumSides=3  GraphicOpacity=1.0  PolygonOuterRadius=1  PolygonOuterRadiusUnits=m  ProductsOfInertia=[0 0 0]  ProductsOfInertiaUnits=kg*m^2  GraphicShininess=75  GraphicSpecularColor=[0.5 0.5 0.5 1.0]  GraphicVisPropType=SimpleVisualProperties
  Right Bracket : sm_lib/Body Elements/Extruded Solid  GraphicAmbientColor=[0.15 0.15 0.15 1.0]  BasedOnType=Density  CenterOfMass=[0 0 0]  CenterOfMassUnits=m  GraphicDiffuseColor=bracketColor  ExportConvexHullGeometry=off  ExtrusionCrossSection=bracketPoints  ExtrusionCrossSectionUnits=m  Density=rhoBracket  DensityUnits=kg/(m^3)  DoExposeReferenceFrame=on  GraphicEmissiveColor=[0.0 0.0 0.0 1.0]  ExportEntireGeometry=off  ExtrusionLength=Tbracket  ExtrusionLengthUnits=m  ExtrusionType=General  SerializedFrames=<Frames/>  MarkerShape=Sphere  MarkerSize=10  GraphicType=FromGeometry  InertiaType=CalculateFromGeometry  Mass=1  MassUnits=kg  MomentsOfInertia=[1 1 1]  MomentsOfInertiaUnits=kg*m^2  PolygonNumSides=3  GraphicOpacity=1.0  PolygonOuterRadius=1  PolygonOuterRadiusUnits=m  ProductsOfInertia=[0 0 0]  ProductsOfInertiaUnits=kg*m^2  GraphicShininess=75  GraphicSpecularColor=[0.5 0.5 0.5 1.0]  GraphicVisPropType=SimpleVisualProperties
  Base Center : PMIOPort  Side=Left
  Hole Center : PMIOPort  Port=2  Side=Right
  connections:
  Base Cebter to Hole XForm/RConn1 -- Hole Center/RConn1
  Base Center to Right Bracket XForm/RConn1 -- Right Bracket/RConn1
  Base Center to Left Bracket XForm/LConn1 -- Base Center to Right Bracket XForm/LConn1 -- Base Center Frame/RConn1 -- Base Center/RConn1 -- Base Cebter to Hole XForm/LConn1
  Base Center to Left Bracket XForm/RConn1 -- Left Bracket/RConn1

== system sm_carousel_lib/CHS ==
  CHS : sm_lib/Body Elements/Extruded Solid  GraphicAmbientColor=[0.15 0.15 0.15 1.0]  BasedOnType=Density  CenterOfMass=[0 0 0]  CenterOfMassUnits=m  GraphicDiffuseColor=PinColor  ExportConvexHullGeometry=off  ExtrusionCrossSection=Pin  ExtrusionCrossSectionUnits=m  Density=rhoPin  DensityUnits=kg/(m^3)  DoExposeReferenceFrame=on  GraphicEmissiveColor=[0.0 0.0 0.0 1.0]  ExportEntireGeometry=off  ExtrusionLength=PinDepth  ExtrusionLengthUnits=m  ExtrusionType=General  SerializedFrames=<Frames/>  MarkerShape=Sphere  MarkerSize=10  GraphicType=FromGeometry  InertiaType=CalculateFromGeometry  Mass=1  MassUnits=kg  MomentsOfInertia=[1 1 1]  MomentsOfInertiaUnits=kg*m^2  PolygonNumSides=3  GraphicOpacity=1.0  PolygonOuterRadius=1  PolygonOuterRadiusUnits=m  ProductsOfInertia=[0 0 0]  ProductsOfInertiaUnits=kg*m^2  GraphicShininess=75  GraphicSpecularColor=[0.5 0.5 0.5 1.0]  GraphicVisPropType=SimpleVisualProperties
  Center to End XForm : sm_lib/Frames and Transforms/Rigid Transform  TranslationMethod=StandardAxis  TranslationStandardOffset=PinDepth/2  TranslationLengthUnit=m  TranslationStandardAxis=-Z  TranslationCartesianOffset=[0 0 0]  TranslationROffset=0  TranslationROffsetUnits=m  TranslationZOffset=0  TranslationZOffsetUnits=m  TranslationThetaOffset=0  TranslationThetaOffsetUnits=deg  RotationMethod=None  RotationAngleUnits=deg  RotationStandardAxis=+Z  RotationAngle=0  RotationArbitraryAxis=[0 0 1]  FollAlignAxisA=+X  BaseAlignAxisA=+Y  FollAlignAxisB=+Y  BaseAlignAxisB=+Z  RotationSequenceAxes=FollowerAxes  RotationSequence=XYX  RotationSequenceAngles=[0 0 0]  RotationSequenceAnglesUnits=deg  RotationMatrix=[1 0 0; 0 1 0; 0 0 1]
  End Center : PMIOPort  Side=Left
  Middle Center : PMIOPort  Port=2  Side=Right
  connections:
  CHS/RConn1 -- Center to End XForm/LConn1 -- Middle Center/RConn1
  Center to End XForm/RConn1 -- End Center/RConn1

== system sm_carousel_lib/Cab Assembly ==
  Cab Body : $bdroot/Cab Body  CabLength=CabLength  CabWidth=CabWidth  PlateThickness=CabPlateThickness  ConnectorWidth=CabBodyConnW  ConnectorHeight=CabBodyConnH  SpacerHeight=CabWindowHeight  SpacerThickness=SpacerThickness  TubDepth=CabTubDepth  RP_CD=RP_CD  RP_W=RP_W  RP_H=RP_H  RP_TL=RP_TL  RP_HR=RP_HR  RP_PT=RP_PT  RP_HO=RP_HO  rhoCab=rhoCab  CabColor=CabColor
  Dummy : $bdroot/Dummy  height=DummyHeight  personDensity=DummyDensity
  Cab Connection : PMIOPort  Side=Left
  connections:
  Cab Body/RConn1 -- Dummy/LConn1
  Cab Connection/RConn1 -- Cab Body/LConn1

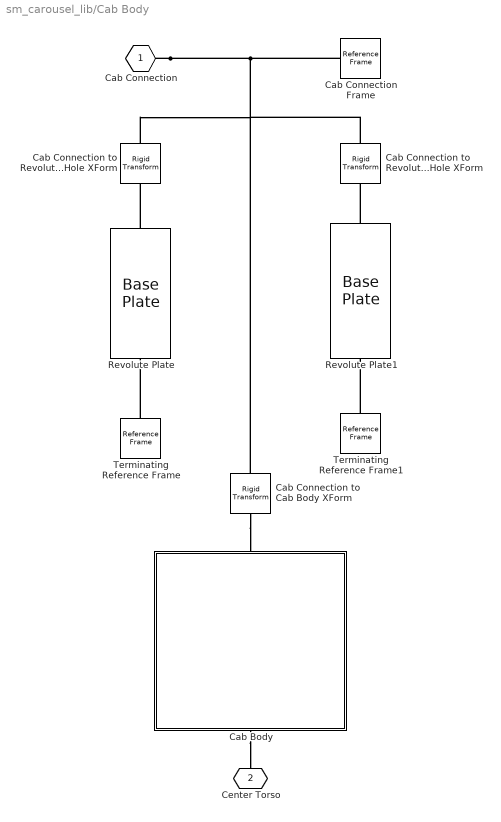
== system sm_carousel_lib/Cab Body ==
  Cab Body : Subsystem
      mask Display:
      | image(fullfile(matlabroot,'toolbox','physmod','sm','smdemos','carousel','images','sm_carousel_cab_main.png'));
      | port_label('lconn',1,'CC');
      | port_label('rconn',1,'CT');
  Cab Connection Frame : sm_lib/Frames and Transforms/Reference Frame
  Cab Connection to Cab Body XForm : sm_lib/Frames and Transforms/Rigid Transform  TranslationMethod=Cartesian  TranslationStandardOffset=0  TranslationLengthUnit=m  TranslationStandardAxis=+Z  TranslationCartesianOffset=CabConnectorOffsetFromPlate  TranslationROffset=0  TranslationROffsetUnits=m  TranslationZOffset=0  TranslationZOffsetUnits=m  TranslationThetaOffset=0  TranslationThetaOffsetUnits=deg  RotationMethod=AlignedAxes  RotationAngleUnits=deg  RotationStandardAxis=+Z  RotationAngle=0  RotationArbitraryAxis=[0 0 1]  FollAlignAxisA=+Z  BaseAlignAxisA=+X  FollAlignAxisB=+X  BaseAlignAxisB=+Z  RotationSequenceAxes=FollowerAxes  RotationSequence=XYX  RotationSequenceAngles=[0 0 0]  RotationSequenceAnglesUnits=deg  RotationMatrix=[1 0 0; 0 1 0; 0 0 1]
  Cab Connection to Revolute Plate1 Hole XForm : sm_lib/Frames and Transforms/Rigid Transform  TranslationMethod=StandardAxis  TranslationStandardOffset=CabRotatePlateOffset  TranslationLengthUnit=m  TranslationStandardAxis=-Z  TranslationCartesianOffset=[0 0 0]  TranslationROffset=0  TranslationROffsetUnits=m  TranslationZOffset=0  TranslationZOffsetUnits=m  TranslationThetaOffset=0  TranslationThetaOffsetUnits=deg  RotationMethod=None  RotationAngleUnits=deg  RotationStandardAxis=+Z  RotationAngle=0  RotationArbitraryAxis=[0 0 1]  FollAlignAxisA=+X  BaseAlignAxisA=+Y  FollAlignAxisB=+Y  BaseAlignAxisB=+Z  RotationSequenceAxes=FollowerAxes  RotationSequence=XYX  RotationSequenceAngles=[0 0 0]  RotationSequenceAnglesUnits=deg  RotationMatrix=[1 0 0; 0 1 0; 0 0 1]
  Cab Connection to Revolute Plate Hole XForm : sm_lib/Frames and Transforms/Rigid Transform  TranslationMethod=StandardAxis  TranslationStandardOffset=CabRotatePlateOffset  TranslationLengthUnit=m  TranslationStandardAxis=+Z  TranslationCartesianOffset=[0 0 0]  TranslationROffset=0  TranslationROffsetUnits=m  TranslationZOffset=0  TranslationZOffsetUnits=m  TranslationThetaOffset=0  TranslationThetaOffsetUnits=deg  RotationMethod=None  RotationAngleUnits=deg  RotationStandardAxis=+Z  RotationAngle=0  RotationArbitraryAxis=[0 0 1]  FollAlignAxisA=+X  BaseAlignAxisA=+Y  FollAlignAxisB=+Y  BaseAlignAxisB=+Z  RotationSequenceAxes=FollowerAxes  RotationSequence=XYX  RotationSequenceAngles=[0 0 0]  RotationSequenceAnglesUnits=deg  RotationMatrix=[1 0 0; 0 1 0; 0 0 1]
  Revolute Plate : $bdroot/Base Plate  ConnectionDepth=RP_CD  BasePlateWidth=RP_W  BasePlateHeight=RP_H  TaperedLength=RP_TL  rHole=RP_HR  BasePlateThickness=RP_PT  HoleOffset=RP_HO  rho=rhoCab  PlateColor=CabColor
  Revolute Plate1 : $bdroot/Base Plate  ConnectionDepth=RP_CD  BasePlateWidth=RP_W  BasePlateHeight=RP_H  TaperedLength=RP_TL  rHole=RP_HR  BasePlateThickness=RP_PT  HoleOffset=RP_HO  rho=rhoCab  PlateColor=CabColor
  Terminating Reference Frame : sm_lib/Frames and Transforms/Reference Frame
  Terminating Reference Frame1 : sm_lib/Frames and Transforms/Reference Frame
  Cab Connection : PMIOPort  Side=Left
  Center Torso : PMIOPort  Port=2  Side=Right
  connections:
  Cab Connection/RConn1 -- Cab Connection to Cab Body XForm/LConn1 -- Cab Connection to Revolute Plate Hole XForm/LConn1 -- Cab Connection to Revolute Plate1 Hole XForm/LConn1 -- Cab Connection Frame/RConn1
  Cab Body/RConn1 -- Center Torso/RConn1
  Revolute Plate1/RConn1 -- Cab Connection to Revolute Plate1 Hole XForm/RConn1
  Revolute Plate/RConn1 -- Cab Connection to Revolute Plate Hole XForm/RConn1
  Terminating Reference Frame1/RConn1 -- Revolute Plate1/LConn1
  Terminating Reference Frame/RConn1 -- Revolute Plate/LConn1
  Cab Connection to Cab Body XForm/RConn1 -- Cab Body/LConn1
